simulink model "Main_Sfunction_blocks"  (R2022b)
settings: Solver=FixedStepAuto  StartTime=0.0  StopTime=sim_time-0.02  FixedStep=0.005
undefined symbols (not defined in the file): A_d, B_d, bike_params, C1, C2, counter, D1, D2, D_balancing_inner, D_balancing_outer, DWORK0, DWORK1, DWORK2, e1_max, g, hor_dis, I_balancing_inner, I_balancing_outer, Initial_State, initial_state, initial_state_estimate, k1, k2, Kalman_gain1, Kalman_gain2, lambda, lf, lr, P_balancing_inner, P_balancing_outer, Parameters, pert_deltadot_state, pert_deltadot_state_fun, pert_phidot_state, pert_phidot_state_fun, Psiref, ref_dis, ref_start_idx, T, Ts, v, Xref, Yref
libraries: eeGeneralControl x3, slpidlib x2, simulink x2
(part 1 of 2)
settings Model: PauseTimes=0.16  Creator=Hadi Hajieghrary  LastModifiedBy=levi1
settings SolverCC: MaxConsecutiveMinStep=10  ZeroCrossAlgorithm=Adaptive  AlgebraicLoopSolver=TrustRegion  AutoInsertRateTranBlk=on
settings DebuggingCC: AlgebraicLoopMsg=none  UnconnectedInputMsg=warning  UnconnectedOutputMsg=warning  UnconnectedLineMsg=warning
settings ModelReferenceCC: EnableRefExpFcnMdlSchedulingChecks=on
settings RTWCC: GenCodeOnly=on  DLArmComputeVersion=19.05

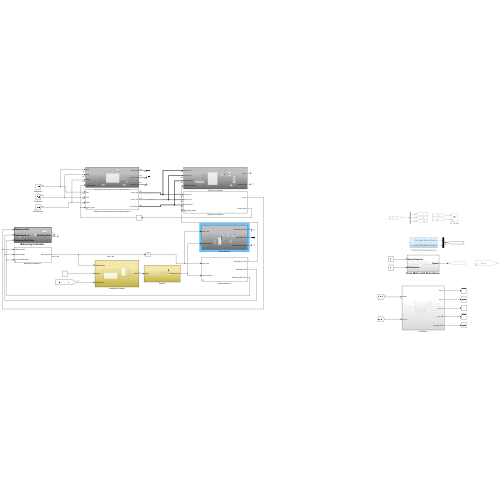
[thumbnail: Simulink's stored preview of the top-level diagram]
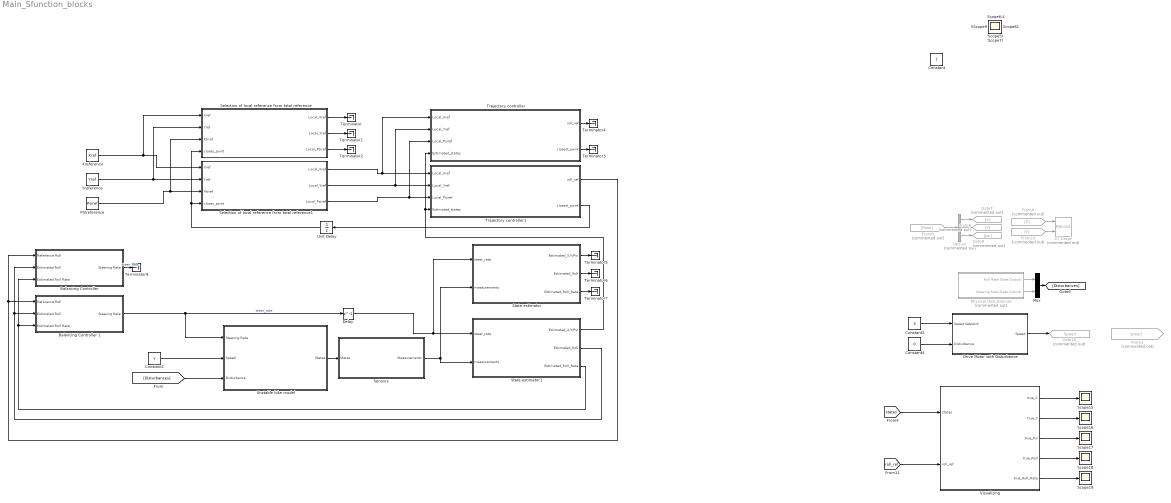
== system Main_Sfunction_blocks ==
  "Balancing Controller " : Subsystem  TreatAsAtomicUnit=on  SystemSampleTime=Ts
      settings: MinAlgLoopOccurrences=on
  Balancing Controller 1 : Subsystem
      mask help: Simulink:masks:GenSFuncDesc_MD
      mask Help: eval('feval(''rtwprivate'',''rtwhelpview'',''rtw_sfcn_block'')');
  Constant1 : Constant  Value=v
  Constant3 : Constant  Value=3
  Constant4 : Constant  Value=0
  Delay : Delay  DelayLength=1  SampleTime=Ts
  Demux : Demux  Commented=on  Outputs=3
  Drive Motor with Disturbance : Subsystem
  From1 : From  Commented=on  GotoTag=Speed  TagVisibility=global
  From10 : From  Commented=on  GotoTag=Y
  From8 : From  Commented=on  GotoTag=Pose
  From9 : From  Commented=on  GotoTag=X
  Goto10 : Goto  Commented=on  GotoTag=Speed  TagVisibility=global
  Goto7 : Goto  Commented=on  GotoTag=X
  Goto8 : Goto  Commented=on  GotoTag=Y
  Goto9 : Goto  Commented=on  GotoTag=psi
  Mux : Mux  Inputs=2
  PSIreference : Constant  Value=Psiref
  Physical Disturbances : Subsystem  Commented=on
  Scope{,1..19} (20 alike) : Scope
  Selection of local reference from total reference : Subsystem
  Selection of local reference from total reference1 : Subsystem
      mask help: Simulink:masks:GenSFuncDesc_MD
      mask Help: eval('feval(''rtwprivate'',''rtwhelpview'',''rtw_sfcn_block'')');
  Sensors : Subsystem
  State estimator : Subsystem
  State estimator1 : Subsystem
      mask help: Simulink:masks:GenSFuncDesc_MD
      mask Help: eval('feval(''rtwprivate'',''rtwhelpview'',''rtw_sfcn_block'')');
  Terminator{,1..8} (9 alike) : Terminator
  Trajectory controller : Subsystem
  Trajectory controller1 : Subsystem
      mask help: Simulink:masks:GenSFuncDesc_MD
      mask Help: eval('feval(''rtwprivate'',''rtwhelpview'',''rtw_sfcn_block'')');
  Unit Delay : UnitDelay  InitialCondition=ref_start_idx  SampleTime=Ts  HasFrameUpgradeWarning=on
  Unstable bike model : Subsystem
  Visualizing : Subsystem
  XY Graph : Record  Commented=on  FileSettingsInternal="{\"entries\":[{\"content\":{\"excelSettings\":{\"content\":{},\"type\":\"Streamout.ExcelSettings\"}},\"type\":\"Streamout.FileSettingStorage\",\"uuid\":\"3eafbd0c-e137-4ee7-8d03-04bb30acaa48\"}],\"packageUris\":[\"http://schema.mathworks.com/mf0/streamout_blocks/R2020a\"],\"version\":\"1.0\"}"  Layout=[1 1]  SignalsInternal="{\"entries\":[{\"content\":{\"signals\":[]},\"type\":\"RecordBlkView.InputSignals\",\"uuid\":\"6eef560f-cd8b-4d38-ad5e-a10ba84618eb\"}],\"packageUris\":[\"http://schema.mathworks.com/mf0/streamout_blocks/R2020a\"],\"version\":\"1.0\"}"  VisualizationBindings="{\"xyplotplugin\":{\"info\":[{\"series\":[],\"subplotID\":1}]}}"  CompatibilityTag=XY
  Xreference : Constant  Value=Xref
  Yreference : Constant  Value=Yref
  Constant : Constant  IOType=siggen
  wires:
  From8/1 -> Demux/1
  Demux/1 -> Goto7/1
  Demux/2 -> Goto8/1
  Demux/3 -> Goto9/1
  From10/1 -> XY Graph/2
  From9/1 -> XY Graph/1
  Physical Disturbances/1(Roll Rate State Disturb) -> Mux/1
  Physical Disturbances/2(Steering Rate State Disturb) -> Mux/2
  Mux/1 -> [Disturbances]
  Drive Motor with Disturbance/1(Speed) -> Goto10/1
  Constant3/1 -> Drive Motor with Disturbance/1(Speed Setpoint)
  Constant4/1 -> Drive Motor with Disturbance/2(Disturbance)
  Balancing Controller 1/1(Steering Rate) -> Unstable bike model/1(Steering Rate), Delay/1  "steer_rate"
  [Disturbances] -> Unstable bike model/3(Disturbance)
  [states] -> Visualizing/1(states)
  Visualizing/1(true_X) -> Scope15/1
  Visualizing/2(true_Y) -> Scope16/1
  Visualizing/3(true_Psi) -> Scope17/1
  Visualizing/4(true_Roll) -> Scope18/1
  Visualizing/5(true_Roll_Rate) -> Scope19/1
  [roll_ref] -> Visualizing/2(roll_ref)
  Unstable bike model/1(States) -> Sensors/1(States)
  Constant1/1 -> Unstable bike model/2(Speed)
  Xreference/1 -> Selection of local reference from total reference/1(Xref), Selection of local reference from total reference1/1(Xref)
  Yreference/1 -> Selection of local reference from total reference/2(Yref), Selection of local reference from total reference1/2(Yref)
  PSIreference/1 -> Selection of local reference from total reference/3(Psiref), Selection of local reference from total reference1/3(Psiref)
  Selection of local reference from total reference1/1(Local_Xref) -> Trajectory controller/1(Local_Xref), Trajectory controller1/1(Local_Xref)
  Selection of local reference from total reference1/2(Local_Yref) -> Trajectory controller/2(Local_Yref), Trajectory controller1/2(Local_Yref)
  Selection of local reference from total reference1/3(Local_Psiref) -> Trajectory controller/3(Local_Psiref), Trajectory controller1/3(Local_Psiref)
  Trajectory controller1/2(closest_point) -> Unit Delay/1
  Unit Delay/1 -> Selection of local reference from total reference/4(closes_point), Selection of local reference from total reference1/4(closes_point)
  Trajectory controller1/1(roll_ref) -> "Balancing Controller "/1(Reference Roll), Balancing Controller 1/1(Reference Roll)
  Sensors/1(Measurements) -> State estimator1/2(measurements), State estimator/2(measurements)
  Delay/1 -> State estimator1/1(steer_rate), State estimator/1(steer_rate)
  State estimator1/1(Estimated_X/Y/Psi) -> Trajectory controller/4(Estimated_states), Trajectory controller1/4(Estimated_states)
  State estimator1/2(Estimated_Roll) -> "Balancing Controller "/2(Estimated Roll), Balancing Controller 1/2(Estimated Roll)
  State estimator1/3(Estimated_Roll_Rate) -> "Balancing Controller "/3(Estimated Roll Rate), Balancing Controller 1/3(Estimated Roll Rate)
  Selection of local reference from total reference/1(Local_Xref) -> Terminator/1
  Selection of local reference from total reference/3(Local_Psiref) -> Terminator2/1
  Selection of local reference from total reference/2(Local_Yref) -> Terminator1/1
  Trajectory controller/1(roll_ref) -> Terminator4/1
  Trajectory controller/2(closest_point) -> Terminator3/1
  State estimator/1(Estimated_X/Y/Psi) -> Terminator5/1
  State estimator/3(Estimated_Roll_Rate) -> Terminator7/1
  State estimator/2(Estimated_Roll) -> Terminator6/1
  "Balancing Controller "/1(Steering Rate) -> Terminator8/1  "steer_rate"

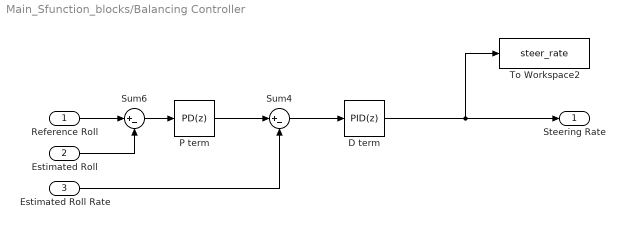
== system Main_Sfunction_blocks/Balancing Controller  ==
  Reference Roll : Inport
  Estimated Roll : Inport  Port=2
  Estimated Roll Rate : Inport  Port=3
  D term : slpidlib/PID Controller  Controller=PID  Form=Parallel  TimeDomain=Discrete-time  UseExternalTs=off  SampleTime=Ts  IntegratorMethod=Forward Euler  FilterMethod=Forward Euler  ControllerParametersSource=internal  P=P_balancing_inner  I=I_balancing_inner  UseKiTs=off  D=D_balancing_inner  N=100  UseFilter=off  TunerSelectOption=Transfer Function Based (PID Tuner App)  InitialConditionSource=internal  InitialConditionForIntegrator=0  InitialConditionForFilter=0  DifferentiatorICPrevScaledInput=0  ExternalReset=none  TrackingMode=off  Kt=1  LimitOutput=off  SatLimitsSource=internal  UpperSaturationLimit=inf  LowerSaturationLimit=-inf  LinearizeAsGain=on  AntiWindupMode=none  Kb=1  LimitIntegrator=off  UpperIntegratorSaturationLimit=inf  LowerIntegratorSaturationLimit=-inf  POutMin=[]  POutMax=[]  IOutMin=[]  IOutMax=[]  DOutMin=[]  DOutMax=[]  NOutMin=[]  NOutMax=[]  SumOutMin=[]  SumOutMax=[]  SaturationOutMin=[]  SaturationOutMax=[]  PParamMin=[]  PParamMax=[]  IParamMin=[]  IParamMax=[]  DParamMin=[]  DParamMax=[]  NParamMin=[]  NParamMax=[]  KbParamMin=[]  KbParamMax=[]  KtParamMin=[]  KtParamMax=[]  KbOutMin=[]  KbOutMax=[]  KtOutMin=[]  KtOutMax=[]  IntegratorOutMin=[]  IntegratorOutMax=[]  FilterOutMin=[]  FilterOutMax=[]  SumI1OutMin=[]  SumI1OutMax=[]  SumI2OutMin=[]  SumI2OutMax=[]  SumI3OutMin=[]  SumI3OutMax=[]  SumI4OutMin=[]  SumI4OutMax=[]  SumDOutMin=[]  SumDOutMax=[]  DifferentiatorOutMin=[]  DifferentiatorOutMax=[]  FilterDiffOutCoefMin=[]  FilterDiffOutCoefMax=[]  ReciprocalOutMin=[]  ReciprocalOutMax=[]  SumDenOutMin=[]  SumDenOutMax=[]  SumNumOutMin=[]  SumNumOutMax=[]  DivideOutMin=[]  DivideOutMax=[]  UdiffTsProdOutMin=[]  UdiffTsProdOutMax=[]  NTsProdOutMin=[]  NTsProdOutMax=[]  UintegralTsProdOutMin=[]  UintegralTsProdOutMax=[]  UngainTsProdOutMin=[]  UngainTsProdOutMax=[]  IntegratorContinuousStateAttributes=''  IntegratorStateMustResolveToSignalObject=off  IntegratorRTWStateStorageClass=Auto  FilterContinuousStateAttributes=''  FilterStateMustResolveToSignalObject=off  FilterRTWStateStorageClass=Auto  ParallelPVariant=InternalParameters  IdealPVariant=Disabled  IVariant=InternalParameters  DVariant=InternalParameters  IntegratorVariant=Discrete  SatVariant=Disabled  AWVariant=Passthrough  PCopyVariant=Disabled  TRVariant=Disabled  FdbkBlocksVariant=Forward  IdealPFdbkVariant=Disabled  SatFdbkVariant=Disabled  DerivativeFilterVariant=Differentiator  NVariant=Passthrough  NCopyVariant=Disabled_SignalSpec  FilterICVariant=InternalICsDifferentiator  IntegratorICVariant=InternalICs  ExternalResetVariant=Disabled  TRSumVariant=Passthrough  SumFdbkVariant=Disabled  SumVariant=Sum_PID  TsampFilterVariant=InternalTs  TsampNgainVariant=Passthrough  TsampIntegralVariant=Passthrough  ExternalSaturationOutDataTypeStr=Inherit: Same as second input
  P term : slpidlib/PID Controller  Controller=PD  Form=Parallel  TimeDomain=Discrete-time  UseExternalTs=off  SampleTime=Ts  IntegratorMethod=Forward Euler  FilterMethod=Forward Euler  ControllerParametersSource=internal  P=P_balancing_outer  I=I_balancing_outer  UseKiTs=off  D=D_balancing_outer  N=100  UseFilter=off  TunerSelectOption=Transfer Function Based (PID Tuner App)  InitialConditionSource=internal  InitialConditionForIntegrator=0  InitialConditionForFilter=0  DifferentiatorICPrevScaledInput=0  ExternalReset=none  TrackingMode=off  Kt=1  LimitOutput=off  SatLimitsSource=internal  UpperSaturationLimit=inf  LowerSaturationLimit=-inf  LinearizeAsGain=on  AntiWindupMode=none  Kb=1  LimitIntegrator=off  UpperIntegratorSaturationLimit=inf  LowerIntegratorSaturationLimit=-inf  POutMin=[]  POutMax=[]  IOutMin=[]  IOutMax=[]  DOutMin=[]  DOutMax=[]  NOutMin=[]  NOutMax=[]  SumOutMin=[]  SumOutMax=[]  SaturationOutMin=[]  SaturationOutMax=[]  PParamMin=[]  PParamMax=[]  IParamMin=[]  IParamMax=[]  DParamMin=[]  DParamMax=[]  NParamMin=[]  NParamMax=[]  KbParamMin=[]  KbParamMax=[]  KtParamMin=[]  KtParamMax=[]  KbOutMin=[]  KbOutMax=[]  KtOutMin=[]  KtOutMax=[]  IntegratorOutMin=[]  IntegratorOutMax=[]  FilterOutMin=[]  FilterOutMax=[]  SumI1OutMin=[]  SumI1OutMax=[]  SumI2OutMin=[]  SumI2OutMax=[]  SumI3OutMin=[]  SumI3OutMax=[]  SumI4OutMin=[]  SumI4OutMax=[]  SumDOutMin=[]  SumDOutMax=[]  DifferentiatorOutMin=[]  DifferentiatorOutMax=[]  FilterDiffOutCoefMin=[]  FilterDiffOutCoefMax=[]  ReciprocalOutMin=[]  ReciprocalOutMax=[]  SumDenOutMin=[]  SumDenOutMax=[]  SumNumOutMin=[]  SumNumOutMax=[]  DivideOutMin=[]  DivideOutMax=[]  UdiffTsProdOutMin=[]  UdiffTsProdOutMax=[]  NTsProdOutMin=[]  NTsProdOutMax=[]  UintegralTsProdOutMin=[]  UintegralTsProdOutMax=[]  UngainTsProdOutMin=[]  UngainTsProdOutMax=[]  IntegratorContinuousStateAttributes=''  IntegratorStateMustResolveToSignalObject=off  IntegratorRTWStateStorageClass=Auto  FilterContinuousStateAttributes=''  FilterStateMustResolveToSignalObject=off  FilterRTWStateStorageClass=Auto  ParallelPVariant=InternalParameters  IdealPVariant=Disabled  IVariant=Disabled  DVariant=InternalParameters  IntegratorVariant=Disabled  SatVariant=Disabled  AWVariant=Disabled  PCopyVariant=Disabled  TRVariant=Disabled  FdbkBlocksVariant=Forward  IdealPFdbkVariant=Disabled  SatFdbkVariant=Disabled  DerivativeFilterVariant=Differentiator  NVariant=Passthrough  NCopyVariant=Disabled_SignalSpec  FilterICVariant=InternalICsDifferentiator  IntegratorICVariant=Disabled  ExternalResetVariant=Disabled  TRSumVariant=Passthrough  SumFdbkVariant=Disabled  SumVariant=Sum_PD  TsampFilterVariant=InternalTs  TsampNgainVariant=Passthrough  TsampIntegralVariant=Disabled_SignalSpec  ExternalSaturationOutDataTypeStr=Inherit: Same as second input
  Sum4 : Sum  Inputs=|+-
  Sum6 : Sum  Inputs=|+-
  To Workspace2 : ToWorkspace  VariableName=steer_rate  SaveFormat=Timeseries  SampleTime=-1
  Steering Rate : Outport
  wires:
  Sum4/1 -> D term/1
  Reference Roll/1 -> Sum6/1
  Sum6/1 -> P term/1
  Estimated Roll Rate/1 -> Sum4/2
  P term/1 -> Sum4/1
  D term/1 -> To Workspace2/1, Steering Rate/1
  Estimated Roll/1 -> Sum6/2

== system Main_Sfunction_blocks/Balancing Controller 1 ==
  Reference Roll : Inport
  Estimated Roll : Inport  Port=2
  Estimated Roll Rate : Inport  Port=3
  Balancing Controller _sfcn : S-Function  FunctionName=Balancing_sf  SFunctionModules=""  SFunctionDeploymentMode=off  EnableBusSupport=off  SFcnStateName=DWORK0,DWORK1,DWORK2  mask{rtw_sf_name=Balancing_sf, showVar=off}
      mask prompts: rtw_sf_name "Simulink:masks:GenSFuncName_MP"; showVar "Simulink:masks:GenSFuncShowModuleList_MP"
      mask help: Simulink:masks:GenSFuncDesc_MD
      mask init:
      | displist = '';
      | if ~strcmp(get_param(gcb, 'FunctionName'), rtw_sf_name);
      |   set_param(gcb, 'FunctionName', rtw_sf_name);
      | end
      | % Check if we are generating code
      | rtw_mode = false;
      | if strcmpi(get_param(bdroot(gcb),'SimulationStatus'),'Initializing')
      | 	rtw_mode = strcmpi(get_param(bdroot(gcb),'BuildingRTWCode'),'on') && ...
      | 		~strcmpi(get_param(bdroot(gcb),'TargetStyle'),'SimulationTarget');
      | end
      | if showVar || rtw_mode
      | 	if exist('rtwsfunc') == 2 | exist('rtwsfunc') == 6
      | 		tmplist = rtwsfunc(rtw_sf_name,gcb);
      | 		tmplist = DAStudio.message('Simulink:masks:GenSFuncListOfModules_IC', tmplist);
      | 	elseif showVar
      | 		tmplist1 = DAStudio.message('Simulink:masks:GenSFuncListOfModules_IC', '');
      |         tmplist2 = DAStudio.message('Simulink:masks:GenSFuncNotLicensed_IC');
      |         tmplist = [tmplist1 tmplist2];
      |  	end
      | end
      | if showVar
      |   displist = tmplist;
      | end
      settings: SFcnIsStateOwnerBlock=on
      settings: CopyFcn=|
      | if ~strcmp(get_param(gcb,'Linkstatus'),'none') && ...
      | ~strcmp(get_param(gcb,'Linkstatus'),'implicit')
      |   set_param(gcb,'LinkStatus','none');
      | end
      mask Help: eval('feval(''rtwprivate'',''rtwhelpview'',''rtw_sfcn_block'')');
      mask Display:
      | port_label('input',1,'Reference Roll');
      | port_label('input',2,'Estimated Roll');
      | port_label('input',3,'Estimated Roll Rate');
      | port_label('output',1,'Steering Rate');
  __InputSSForSFun__ : Subsystem
  __OutputSSForSFun__ : Subsystem
  Steering Rate : Outport
  wires:
  __OutputSSForSFun__/1(Steering Rate) -> Steering Rate/1
  Balancing Controller _sfcn/1 -> __OutputSSForSFun__/1(__UniqueInportName__1__)
  __InputSSForSFun__/3(__UniqueOutportName__3__) -> Balancing Controller _sfcn/3
  __InputSSForSFun__/2(__UniqueOutportName__2__) -> Balancing Controller _sfcn/2
  __InputSSForSFun__/1(__UniqueOutportName__1__) -> Balancing Controller _sfcn/1
  Estimated Roll Rate/1 -> __InputSSForSFun__/3(Estimated Roll Rate)
  Estimated Roll/1 -> __InputSSForSFun__/2(Estimated Roll)
  Reference Roll/1 -> __InputSSForSFun__/1(Reference Roll)

== system Main_Sfunction_blocks/Drive Motor with Disturbance ==
  Speed Setpoint : Inport
  Disturbance : Inport  Port=2
  Sum2 : Sum  Inputs=++|
  Transfer Fcn : TransferFcn  Denominator=[2 1]
  Speed : Outport
  wires:
  Sum2/1 -> Speed/1
  Transfer Fcn/1 -> Sum2/2
  Speed Setpoint/1 -> Transfer Fcn/1
  Disturbance/1 -> Sum2/1

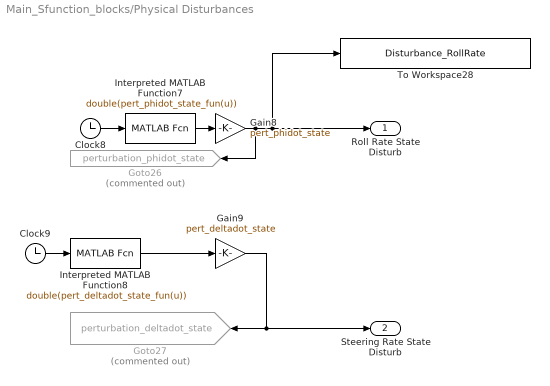
== system Main_Sfunction_blocks/Physical Disturbances ==
  Clock8 : Clock
  Clock9 : Clock
  Gain8 : Gain  Gain=pert_phidot_state
  Gain9 : Gain  Gain=pert_deltadot_state
  Goto26 : Goto  Commented=on  GotoTag=perturbation_phidot_state  TagVisibility=global
  Goto27 : Goto  Commented=on  GotoTag=perturbation_deltadot_state  TagVisibility=global
  Interpreted MATLAB Function7 : MATLABFcn  MATLABFcn=double(pert_phidot_state_fun(u))
  Interpreted MATLAB Function8 : MATLABFcn  MATLABFcn=double(pert_deltadot_state_fun(u))
  To Workspace28 : ToWorkspace  VariableName=Disturbance_RollRate  SaveFormat=Timeseries  SampleTime=-1
  Roll Rate State Disturb : Outport
  Steering Rate State Disturb : Outport  Port=2
  wires:
  Interpreted MATLAB Function7/1 -> Gain8/1
  Clock8/1 -> Interpreted MATLAB Function7/1
  Gain8/1 -> Goto26/1, Roll Rate State Disturb/1, To Workspace28/1
  Interpreted MATLAB Function8/1 -> Gain9/1
  Clock9/1 -> Interpreted MATLAB Function8/1
  Gain9/1 -> Steering Rate State Disturb/1, Goto27/1

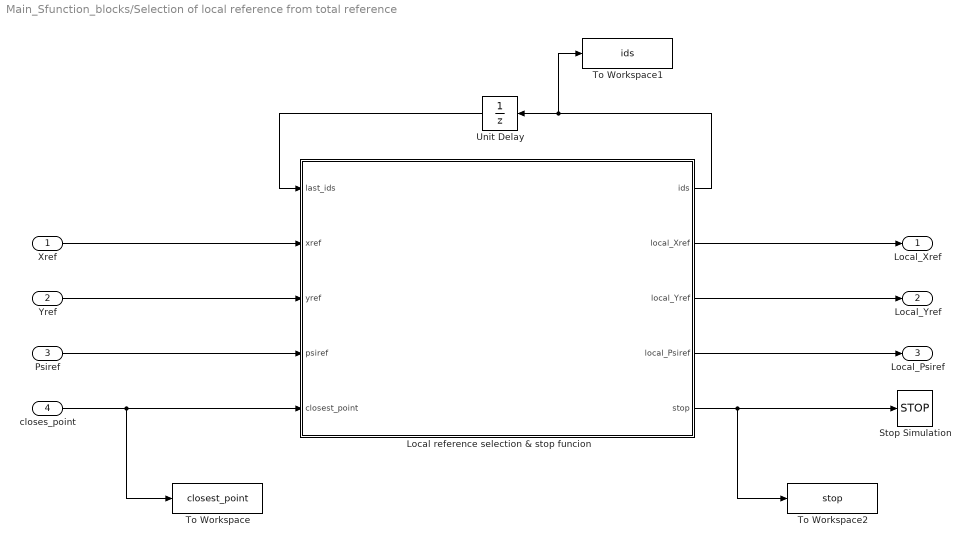
== system Main_Sfunction_blocks/Selection of local reference from total reference ==
  Xref : Inport
  Yref : Inport  Port=2
  Psiref : Inport  Port=3
  closes_point : Inport  Port=4
  Local reference selection & stop funcion : MATLAB Function  TreatAsAtomicUnit=on
  Stop Simulation : Stop
  To Workspace : ToWorkspace  VariableName=closest_point  SaveFormat=Timeseries  SampleTime=-1
  To Workspace1 : ToWorkspace  VariableName=ids  SaveFormat=Timeseries  SampleTime=-1
  To Workspace2 : ToWorkspace  VariableName=stop  SaveFormat=Timeseries  SampleTime=-1
  Unit Delay : UnitDelay  InitialCondition=1  SampleTime=Ts  HasFrameUpgradeWarning=on
  Local_Xref : Outport
  Local_Yref : Outport  Port=2
  Local_Psiref : Outport  Port=3
  wires:
  Local reference selection & stop funcion/1(ids) -> To Workspace1/1, Unit Delay/1
  Unit Delay/1 -> Local reference selection & stop funcion/1(last_ids)
  closes_point/1 -> To Workspace/1, Local reference selection & stop funcion/5(closest_point)
  Xref/1 -> Local reference selection & stop funcion/2(xref)
  Yref/1 -> Local reference selection & stop funcion/3(yref)
  Psiref/1 -> Local reference selection & stop funcion/4(psiref)
  Local reference selection & stop funcion/5(stop) -> To Workspace2/1, Stop Simulation/1
  Local reference selection & stop funcion/2(local_Xref) -> Local_Xref/1
  Local reference selection & stop funcion/3(local_Yref) -> Local_Yref/1
  Local reference selection & stop funcion/4(local_Psiref) -> Local_Psiref/1

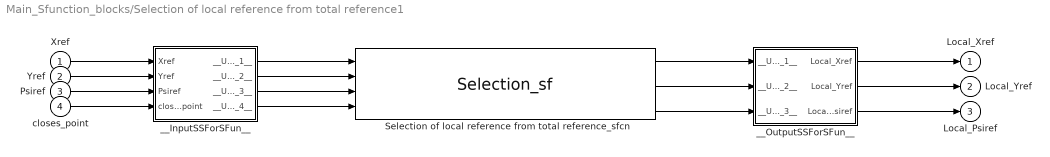
== system Main_Sfunction_blocks/Selection of local reference from total reference1 ==
  Xref : Inport
  Yref : Inport  Port=2
  Psiref : Inport  Port=3
  closes_point : Inport  Port=4
  Selection of local reference from total reference_sfcn : S-Function  FunctionName=Selection_sf  SFunctionModules=""  SFunctionDeploymentMode=off  EnableBusSupport=off  SFcnStateName=DWORK0  mask{rtw_sf_name=Selection_sf, showVar=off}
      mask prompts: rtw_sf_name "Simulink:masks:GenSFuncName_MP"; showVar "Simulink:masks:GenSFuncShowModuleList_MP"
      mask help: Simulink:masks:GenSFuncDesc_MD
      mask init: same as Main_Sfunction_blocks/Balancing Controller 1/Balancing Controller _sfcn
      settings: SFcnIsStateOwnerBlock=on
      settings: CopyFcn=|
      | if ~strcmp(get_param(gcb,'Linkstatus'),'none') && ...
      | ~strcmp(get_param(gcb,'Linkstatus'),'implicit')
      |   set_param(gcb,'LinkStatus','none');
      | end
      mask Help: eval('feval(''rtwprivate'',''rtwhelpview'',''rtw_sfcn_block'')');
      mask Display:
      | port_label('input',1,'Xref');
      | port_label('input',2,'Yref');
      | port_label('input',3,'Psiref');
      | port_label('input',4,'closes_point');
      | port_label('output',1,'Local_Xref');
      | port_label('output',2,'Local_Yref');
      | port_label('output',3,'Local_Psiref');
  __InputSSForSFun__ : Subsystem
  __OutputSSForSFun__ : Subsystem
  Local_Xref : Outport
  Local_Yref : Outport  Port=2
  Local_Psiref : Outport  Port=3
  wires:
  Xref/1 -> __InputSSForSFun__/1(Xref)
  Yref/1 -> __InputSSForSFun__/2(Yref)
  Psiref/1 -> __InputSSForSFun__/3(Psiref)
  closes_point/1 -> __InputSSForSFun__/4(closes_point)
  __InputSSForSFun__/1(__UniqueOutportName__1__) -> Selection of local reference from total reference_sfcn/1
  __InputSSForSFun__/2(__UniqueOutportName__2__) -> Selection of local reference from total reference_sfcn/2
  __InputSSForSFun__/3(__UniqueOutportName__3__) -> Selection of local reference from total reference_sfcn/3
  __InputSSForSFun__/4(__UniqueOutportName__4__) -> Selection of local reference from total reference_sfcn/4
  Selection of local reference from total reference_sfcn/1 -> __OutputSSForSFun__/1(__UniqueInportName__1__)
  Selection of local reference from total reference_sfcn/2 -> __OutputSSForSFun__/2(__UniqueInportName__2__)
  Selection of local reference from total reference_sfcn/3 -> __OutputSSForSFun__/3(__UniqueInportName__3__)
  __OutputSSForSFun__/1(Local_Xref) -> Local_Xref/1
  __OutputSSForSFun__/2(Local_Yref) -> Local_Yref/1
  __OutputSSForSFun__/3(Local_Psiref) -> Local_Psiref/1

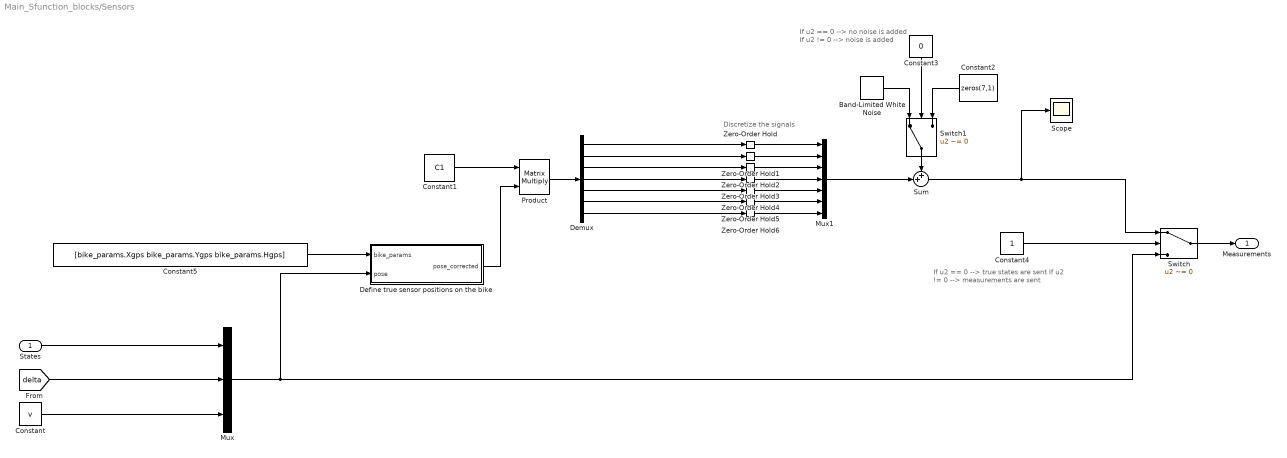
== system Main_Sfunction_blocks/Sensors ==
  note: Discretize the signals
  note: If u2 == 0 --> no noise is added
      | If u2 != 0 --> noise is added
  note: If u2 == 0 --> true states are sent
      | If u2 != 0 --> measurements are sent
  States : Inport
  Band-Limited White Noise : simulink/Sources/Band-Limited White Noise  Cov=ones(7,1)*1e-3  Ts=Ts  seed=[23341]
  Constant : Constant  Value=v
  Constant1 : Constant  Value=C1
  Constant2 : Constant  Value=zeros(7,1)
  Constant3 : Constant  Value=0
  Constant4 : Constant
  Constant5 : Constant  Value=[bike_params.Xgps bike_params.Ygps bike_params.Hgps]
  Define true sensor positions on the bike : MATLAB Function  TreatAsAtomicUnit=on
  Demux : Demux  Outputs=7
  Mux : Mux  Inputs=3
  Mux1 : Mux  Inputs=7
  Product : Product  Multiplication=Matrix(*)
  Scope : Scope
  Sum : Sum  Inputs=++|
  Switch : Switch  Criteria=u2 ~= 0  SaturateOnIntegerOverflow=off  InputSameDT=off
  Switch1 : Switch  Criteria=u2 ~= 0  SaturateOnIntegerOverflow=off  InputSameDT=off
  Zero-Order Hold : ZeroOrderHold  SampleTime=10*Ts
  Zero-Order Hold1 : ZeroOrderHold  SampleTime=10*Ts
  Zero-Order Hold{2..6} (5 alike) : ZeroOrderHold  SampleTime=Ts
  Measurements : Outport
  wires:
  Constant/1 -> Mux/3
  [delta] -> Mux/2
  States/1 -> Mux/1
  Switch/1 -> Measurements/1
  Mux/1 -> Switch/3, Define true sensor positions on the bike/2(pose)
  Constant4/1 -> Switch/2
  Constant1/1 -> Product/1
  Switch1/1 -> Sum/1
  Band-Limited White Noise/1 -> Switch1/1
  Constant2/1 -> Switch1/3
  Constant3/1 -> Switch1/2
  Mux1/1 -> Sum/2
  Product/1 -> Demux/1
  Demux/2 -> Zero-Order Hold1/1
  Demux/3 -> Zero-Order Hold2/1
  Demux/4 -> Zero-Order Hold3/1
  Demux/5 -> Zero-Order Hold4/1
  Demux/6 -> Zero-Order Hold5/1
  Demux/7 -> Zero-Order Hold6/1
  Zero-Order Hold/1 -> Mux1/1
  Zero-Order Hold1/1 -> Mux1/2
  Zero-Order Hold2/1 -> Mux1/3
  Zero-Order Hold3/1 -> Mux1/4
  Zero-Order Hold4/1 -> Mux1/5
  Zero-Order Hold5/1 -> Mux1/6
  Zero-Order Hold6/1 -> Mux1/7
  Sum/1 -> Scope/1, Switch/1
  Demux/1 -> Zero-Order Hold/1
  Define true sensor positions on the bike/1(pose_corrected) -> Product/2
  Constant5/1 -> Define true sensor positions on the bike/1(bike_params)

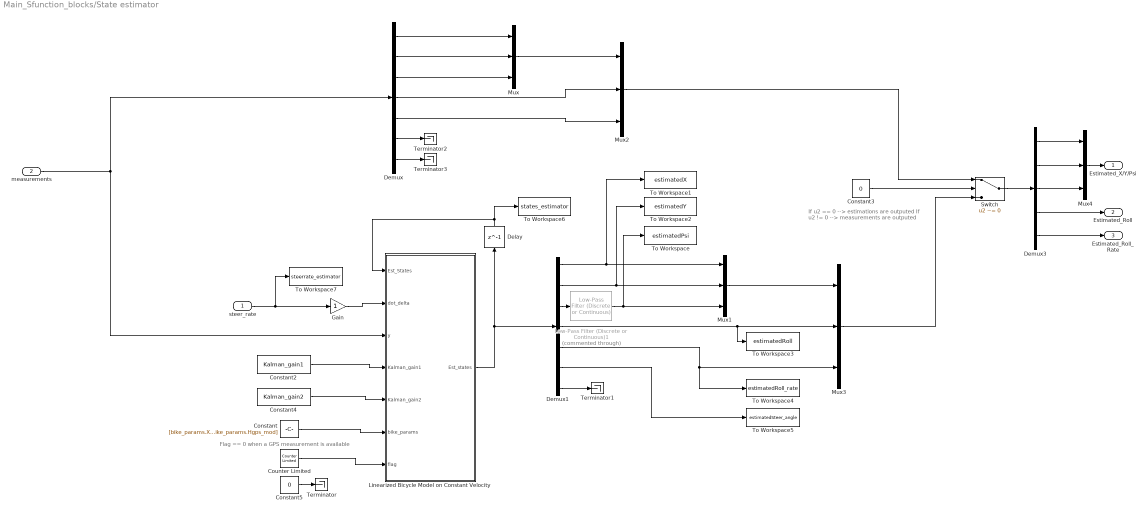
== system Main_Sfunction_blocks/State estimator ==
  note: Flag == 0 when a GPS measurement is available
  note: If u2 == 0 --> estimations are outputed
      | If u2 != 0 --> measurements are outputed
  steer_rate : Inport
  measurements : Inport  Port=2
  Constant : Constant  Value=[bike_params.Xgps_mod bike_params.Ygps_mod bike_params.Hgps_mod]
  Constant2 : Constant  Value=Kalman_gain1  SampleTime=Ts
  Constant3 : Constant  Value=0
  Constant4 : Constant  Value=Kalman_gain2  SampleTime=Ts
  Constant5 : Constant  Value=0
  Counter Limited : simulink/Sources/Counter Limited  uplimit=counter  tsamp=Ts
  Delay : Delay  DelayLength=1  InitialCondition=[initial_state_estimate.x initial_state_estimate.y initial_state_estimate.heading initial_state.roll initial_state.roll_rate initial_state.steering v]  SampleTime=Ts
  Demux : Demux  Outputs=7
  Demux1 : Demux  Outputs=7
  Demux3 : Demux  Outputs=5
  Gain : Gain
  Linearized Bicycle Model on Constant Velocity : MATLAB Function  TreatAsAtomicUnit=on
  Low-Pass Filter (Discrete or Continuous)1 : eeGeneralControl/Low-Pass Filter (Discrete or Continuous)  Commented=through  K=1  T=1  B=inf  A=-inf  init_option=Inherited from block input  x0=0  Ts=Ts
  Mux{,1..4} (5 alike) : Mux  Inputs=3
  Switch : Switch  Criteria=u2 ~= 0  SaturateOnIntegerOverflow=off  InputSameDT=off
  Terminator{,1..3} (4 alike) : Terminator
  To Workspace : ToWorkspace  VariableName=estimatedPsi  SaveFormat=Timeseries  SampleTime=-1
  To Workspace1 : ToWorkspace  VariableName=estimatedX  SaveFormat=Timeseries  SampleTime=-1
  To Workspace2 : ToWorkspace  VariableName=estimatedY  SaveFormat=Timeseries  SampleTime=-1
  To Workspace3 : ToWorkspace  VariableName=estimatedRoll  SaveFormat=Timeseries  SampleTime=-1
  To Workspace4 : ToWorkspace  VariableName=estimatedRoll_rate  SaveFormat=Timeseries  SampleTime=-1
  To Workspace5 : ToWorkspace  VariableName=estimatedSteer_angle  SaveFormat=Timeseries  SampleTime=-1
  To Workspace6 : ToWorkspace  VariableName=states_estimator  SaveFormat=Timeseries  SampleTime=-1
  To Workspace7 : ToWorkspace  VariableName=steerrate_estimator  SaveFormat=Timeseries  SampleTime=-1
  Estimated_X/Y/Psi : Outport  VectorParamsAs1DForOutWhenUnconnected=off
  Estimated_Roll : Outport  Port=2  VectorParamsAs1DForOutWhenUnconnected=off
  Estimated_Roll_Rate : Outport  Port=3  VectorParamsAs1DForOutWhenUnconnected=off
  wires:
  Demux/3 -> Mux/3
  Linearized Bicycle Model on Constant Velocity/1(Est_states) -> Delay/1, Demux1/1
  Gain/1 -> Linearized Bicycle Model on Constant Velocity/2(dot_delta)
  Demux1/6 -> To Workspace5/1
  Demux1/5 -> Mux3/3, To Workspace4/1
  Delay/1 -> Linearized Bicycle Model on Constant Velocity/1(Est_States), To Workspace6/1
  steer_rate/1 -> To Workspace7/1, Gain/1
  Demux1/2 -> To Workspace2/1, Mux1/2
  measurements/1 -> Linearized Bicycle Model on Constant Velocity/3(y), Demux/1
  Demux/1 -> Mux/1
  Demux1/3 -> Low-Pass Filter (Discrete or Continuous)1/1
  Demux1/1 -> Mux1/1, To Workspace1/1
  Demux/2 -> Mux/2
  Demux1/7 -> Terminator1/1
  Demux/7 -> Terminator3/1
  Demux/6 -> Terminator2/1
  Mux/1 -> Mux2/1
  Mux2/1 -> Switch/1
  Mux3/1 -> Switch/3
  Constant3/1 -> Switch/2
  Demux/4 -> Mux2/2
  Demux/5 -> Mux2/3
  Mux1/1 -> Mux3/1
  Demux1/4 -> To Workspace3/1, Mux3/2
  Switch/1 -> Demux3/1
  Demux3/1 -> Mux4/1
  Demux3/2 -> Mux4/2
  Demux3/3 -> Mux4/3
  Mux4/1 -> Estimated_X/Y/Psi/1
  Demux3/4 -> Estimated_Roll/1
  Demux3/5 -> Estimated_Roll_Rate/1
  Constant2/1 -> Linearized Bicycle Model on Constant Velocity/4(Kalman_gain1)
  Constant4/1 -> Linearized Bicycle Model on Constant Velocity/5(Kalman_gain2)
  Counter Limited/1 -> Linearized Bicycle Model on Constant Velocity/7(flag)
  Low-Pass Filter (Discrete or Continuous)1/1 -> To Workspace/1, Mux1/3
  Constant5/1 -> Terminator/1
  Constant/1 -> Linearized Bicycle Model on Constant Velocity/6(bike_params)

== system Main_Sfunction_blocks/State estimator1 ==
  steer_rate : Inport
  measurements : Inport  Port=2
  State estimator_sfcn : S-Function  FunctionName=State_sf  SFunctionModules=""  SFunctionDeploymentMode=off  EnableBusSupport=off  SFcnStateName=DWORK0,DWORK1  mask{rtw_sf_name=State_sf, showVar=off}
      mask prompts: rtw_sf_name "Simulink:masks:GenSFuncName_MP"; showVar "Simulink:masks:GenSFuncShowModuleList_MP"
      mask help: Simulink:masks:GenSFuncDesc_MD
      mask init: same as Main_Sfunction_blocks/Balancing Controller 1/Balancing Controller _sfcn
      settings: SFcnIsStateOwnerBlock=on
      settings: CopyFcn=|
      | if ~strcmp(get_param(gcb,'Linkstatus'),'none') && ...
      | ~strcmp(get_param(gcb,'Linkstatus'),'implicit')
      |   set_param(gcb,'LinkStatus','none');
      | end
      mask Help: eval('feval(''rtwprivate'',''rtwhelpview'',''rtw_sfcn_block'')');
      mask Display:
      | port_label('input',1,'steer_rate');
      | port_label('input',2,'measurements');
      | port_label('output',1,'Estimated_X/Y/Psi');
      | port_label('output',2,'Estimated_Roll');
      | port_label('output',3,'Estimated_Roll_Rate');
  __InputSSForSFun__ : Subsystem
  __OutputSSForSFun__ : Subsystem
  Estimated_X/Y/Psi : Outport  VectorParamsAs1DForOutWhenUnconnected=off
  Estimated_Roll : Outport  Port=2  VectorParamsAs1DForOutWhenUnconnected=off
  Estimated_Roll_Rate : Outport  Port=3  VectorParamsAs1DForOutWhenUnconnected=off
  wires:
  __OutputSSForSFun__/3(Estimated_Roll_Rate) -> Estimated_Roll_Rate/1
  __OutputSSForSFun__/2(Estimated_Roll) -> Estimated_Roll/1
  __OutputSSForSFun__/1(Estimated_X/Y/Psi) -> Estimated_X/Y/Psi/1
  State estimator_sfcn/3 -> __OutputSSForSFun__/3(__UniqueInportName__3__)
  State estimator_sfcn/2 -> __OutputSSForSFun__/2(__UniqueInportName__2__)
  State estimator_sfcn/1 -> __OutputSSForSFun__/1(__UniqueInportName__1__)
  __InputSSForSFun__/2(__UniqueOutportName__2__) -> State estimator_sfcn/2
  __InputSSForSFun__/1(__UniqueOutportName__1__) -> State estimator_sfcn/1
  measurements/1 -> __InputSSForSFun__/2(measurements)
  steer_rate/1 -> __InputSSForSFun__/1(steer_rate)

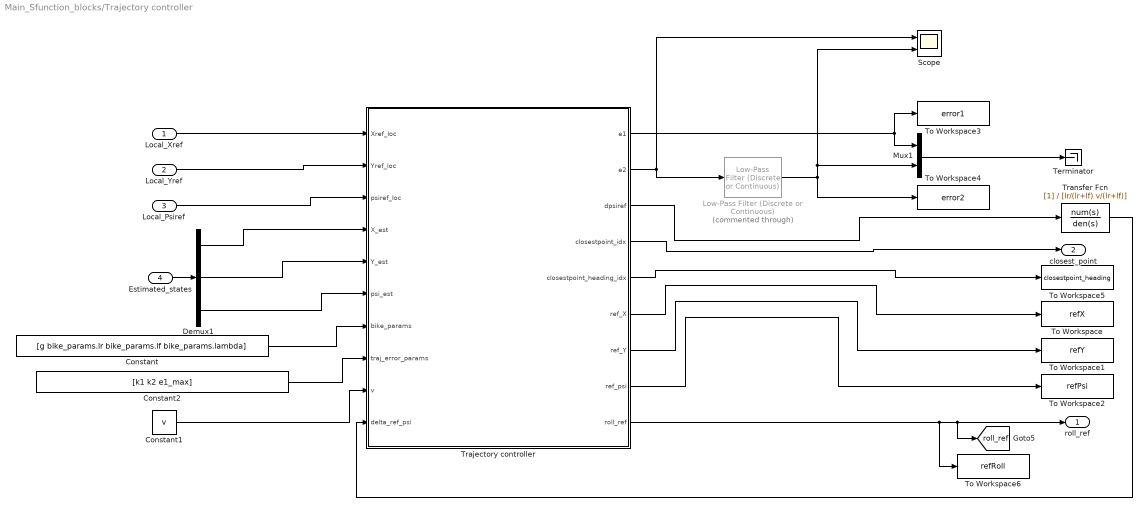
== system Main_Sfunction_blocks/Trajectory controller ==
  Local_Xref : Inport
  Local_Yref : Inport  Port=2
  Local_Psiref : Inport  Port=3
  Estimated_states : Inport  Port=4
  Constant : Constant  Value=[g bike_params.lr bike_params.lf bike_params.lambda]
  Constant1 : Constant  Value=v
  Constant2 : Constant  Value=[k1 k2 e1_max]
  Demux1 : Demux  Outputs=3
  Low-Pass Filter (Discrete or Continuous) : eeGeneralControl/Low-Pass Filter (Discrete or Continuous)  Commented=through  K=1  T=1  B=inf  A=-inf  init_option=Inherited from block input  x0=0  Ts=Ts
  Mux1 : Mux  Inputs=2
  Scope : Scope  NumInputPorts=2
  Terminator : Terminator
  To Workspace : ToWorkspace  VariableName=refX  SaveFormat=Timeseries  SampleTime=-1
  To Workspace1 : ToWorkspace  VariableName=refY  SaveFormat=Timeseries  SampleTime=-1
  To Workspace2 : ToWorkspace  VariableName=refPsi  SaveFormat=Timeseries  SampleTime=-1
  To Workspace3 : ToWorkspace  VariableName=error1  SaveFormat=Timeseries  SampleTime=-1
  To Workspace4 : ToWorkspace  VariableName=error2  SaveFormat=Timeseries  SampleTime=-1
  To Workspace5 : ToWorkspace  VariableName=closestpoint_heading  SaveFormat=Timeseries  SampleTime=-1
  To Workspace6 : ToWorkspace  VariableName=refRoll  SaveFormat=Timeseries  SampleTime=-1
  Trajectory controller : MATLAB Function  TreatAsAtomicUnit=on
  Transfer Fcn : TransferFcn  Denominator=[lr/(lr+lf) v/(lr+lf)]
  roll_ref : Outport
  closest_point : Outport  Port=2
  tag scope: roll_ref=global
  wires:
  Demux1/3 -> Trajectory controller/6(psi_est)
  Trajectory controller/4(closestpoint_idx) -> closest_point/1
  Trajectory controller/5(closestpoint_heading_idx) -> To Workspace5/1
  Estimated_states/1 -> Demux1/1
  Low-Pass Filter (Discrete or Continuous)/1 -> Mux1/2, Scope/2, To Workspace4/1
  Local_Xref/1 -> Trajectory controller/1(Xref_loc)
  Local_Psiref/1 -> Trajectory controller/3(psiref_loc)
  Mux1/1 -> Terminator/1
  Trajectory controller/3(dpsiref) -> Transfer Fcn/1
  Trajectory controller/7(ref_Y) -> To Workspace1/1
  Trajectory controller/2(e2) -> Low-Pass Filter (Discrete or Continuous)/1, Scope/1
  Demux1/2 -> Trajectory controller/5(Y_est)
  Local_Yref/1 -> Trajectory controller/2(Yref_loc)
  Demux1/1 -> Trajectory controller/4(X_est)
  Trajectory controller/6(ref_X) -> To Workspace/1
  Trajectory controller/8(ref_psi) -> To Workspace2/1
  Trajectory controller/1(e1) -> To Workspace3/1, Mux1/1
  Constant1/1 -> Trajectory controller/9(v)
  Constant/1 -> Trajectory controller/7(bike_params)
  Constant2/1 -> Trajectory controller/8(traj_error_params)
  Trajectory controller/9(roll_ref) -> To Workspace6/1, [roll_ref], roll_ref/1
  Transfer Fcn/1 -> Trajectory controller/10(delta_ref_psi)

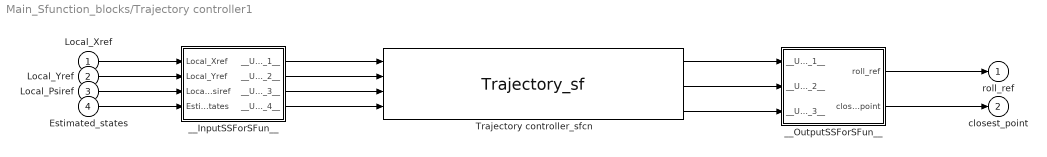
== system Main_Sfunction_blocks/Trajectory controller1 ==
  Local_Xref : Inport
  Local_Yref : Inport  Port=2
  Local_Psiref : Inport  Port=3
  Estimated_states : Inport  Port=4
  Trajectory controller_sfcn : S-Function  FunctionName=Trajectory_sf  SFunctionModules=""  SFunctionDeploymentMode=off  EnableBusSupport=off  mask{rtw_sf_name=Trajectory_sf, showVar=off}
      mask prompts: rtw_sf_name "Simulink:masks:GenSFuncName_MP"; showVar "Simulink:masks:GenSFuncShowModuleList_MP"
      mask help: Simulink:masks:GenSFuncDesc_MD
      mask init: same as Main_Sfunction_blocks/Balancing Controller 1/Balancing Controller _sfcn
      settings: CopyFcn=|
      | if ~strcmp(get_param(gcb,'Linkstatus'),'none') && ...
      | ~strcmp(get_param(gcb,'Linkstatus'),'implicit')
      |   set_param(gcb,'LinkStatus','none');
      | end
      mask Help: eval('feval(''rtwprivate'',''rtwhelpview'',''rtw_sfcn_block'')');
      mask Display:
      | port_label('input',1,'Local_Xref');
      | port_label('input',2,'Local_Yref');
      | port_label('input',3,'Local_Psiref');
      | port_label('input',4,'Estimated_states');
      | port_label('output',1,'roll_ref');
      | port_label('output',2,'closest_point');
      | port_label('output',3,'Outport1');
  __InputSSForSFun__ : Subsystem
  __OutputSSForSFun__ : Subsystem
  roll_ref : Outport
  closest_point : Outport  Port=2
  wires:
  __OutputSSForSFun__/2(closest_point) -> closest_point/1
  __OutputSSForSFun__/1(roll_ref) -> roll_ref/1
  Trajectory controller_sfcn/3 -> __OutputSSForSFun__/3(__UniqueInportName__3__)
  Trajectory controller_sfcn/2 -> __OutputSSForSFun__/2(__UniqueInportName__2__)
  Trajectory controller_sfcn/1 -> __OutputSSForSFun__/1(__UniqueInportName__1__)
  __InputSSForSFun__/4(__UniqueOutportName__4__) -> Trajectory controller_sfcn/4
  __InputSSForSFun__/3(__UniqueOutportName__3__) -> Trajectory controller_sfcn/3
  __InputSSForSFun__/2(__UniqueOutportName__2__) -> Trajectory controller_sfcn/2
  __InputSSForSFun__/1(__UniqueOutportName__1__) -> Trajectory controller_sfcn/1
  Estimated_states/1 -> __InputSSForSFun__/4(Estimated_states)
  Local_Psiref/1 -> __InputSSForSFun__/3(Local_Psiref)
  Local_Yref/1 -> __InputSSForSFun__/2(Local_Yref)
  Local_Xref/1 -> __InputSSForSFun__/1(Local_Xref)

== system Main_Sfunction_blocks/Unstable bike model ==
  Steering Rate : Inport
  Speed : Inport  Port=2
  Disturbance : Inport  Port=3
  Mux : Mux  Inputs=2
  Mux1 : Mux  Inputs=2
  Nonlinear Bicycle model : Subsystem
  Track bycicle pose : Subsystem
  States : Outport
  tag scope: states=global
  wires:
  Steering Rate/1 -> Nonlinear Bicycle model/2(Steering Rate)
  Nonlinear Bicycle model/2(Roll) -> Mux1/1
  Nonlinear Bicycle model/3(Roll Rate) -> Mux1/2
  Mux/1 -> States/1, [states]
  Mux1/1 -> Mux/2
  Speed/1 -> Track bycicle pose/1(Speed), Nonlinear Bicycle model/1(Speed)
  Disturbance/1 -> Nonlinear Bicycle model/3(Disturbances (phi_dot; delta_dot))
  Nonlinear Bicycle model/1(Steer angle) -> Track bycicle pose/2(Steer angle)
  Track bycicle pose/1(Pose) -> Mux/1

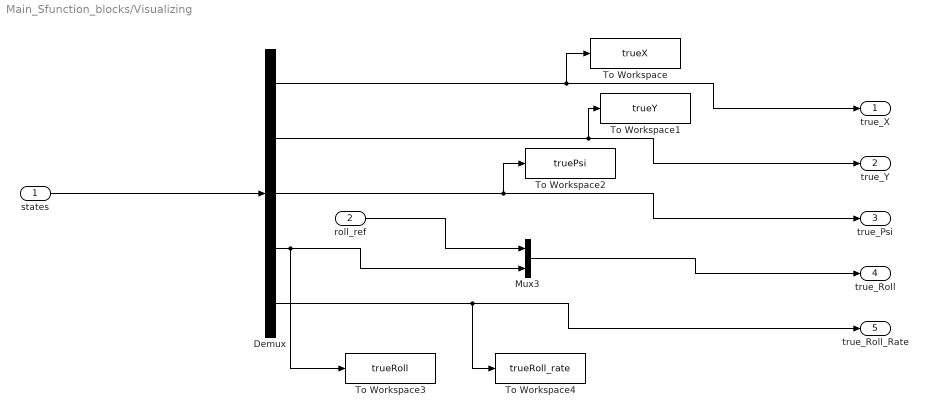
== system Main_Sfunction_blocks/Visualizing ==
  states : Inport
  roll_ref : Inport  Port=2
  Demux : Demux  Outputs=5
  Mux3 : Mux  Inputs=2
  To Workspace : ToWorkspace  VariableName=trueX  SaveFormat=Timeseries  SampleTime=-1
  To Workspace1 : ToWorkspace  VariableName=trueY  SaveFormat=Timeseries  SampleTime=-1
  To Workspace2 : ToWorkspace  VariableName=truePsi  SaveFormat=Timeseries  SampleTime=-1
  To Workspace3 : ToWorkspace  VariableName=trueRoll  SaveFormat=Timeseries  SampleTime=-1
  To Workspace4 : ToWorkspace  VariableName=trueRoll_rate  SaveFormat=Timeseries  SampleTime=-1
  true_X : Outport
  true_Y : Outport  Port=2
  true_Psi : Outport  Port=3
  true_Roll : Outport  Port=4
  true_Roll_Rate : Outport  Port=5
  wires:
  states/1 -> Demux/1
  Demux/1 -> true_X/1, To Workspace/1
  Demux/3 -> To Workspace2/1, true_Psi/1
  roll_ref/1 -> Mux3/1
  Demux/4 -> To Workspace3/1, Mux3/2
  Mux3/1 -> true_Roll/1
  Demux/5 -> To Workspace4/1, true_Roll_Rate/1
  Demux/2 -> To Workspace1/1, true_Y/1

== system Main_Sfunction_blocks/Balancing Controller 1/__InputSSForSFun__ ==
  Reference Roll : Inport
  Estimated Roll : Inport  Port=2
  Estimated Roll Rate : Inport  Port=3
  __UniqueOutportName__1__ : Outport
  __UniqueOutportName__2__ : Outport  Port=2
  __UniqueOutportName__3__ : Outport  Port=3
  wires:
  Estimated Roll Rate/1 -> __UniqueOutportName__3__/1
  Estimated Roll/1 -> __UniqueOutportName__2__/1
  Reference Roll/1 -> __UniqueOutportName__1__/1

== system Main_Sfunction_blocks/Balancing Controller 1/__OutputSSForSFun__ ==
  __UniqueInportName__1__ : Inport
  Steering Rate : Outport
  wires:
  __UniqueInportName__1__/1 -> Steering Rate/1

== system Main_Sfunction_blocks/Selection of local reference from total reference1/__InputSSForSFun__ ==
  Xref : Inport
  Yref : Inport  Port=2
  Psiref : Inport  Port=3
  closes_point : Inport  Port=4
  __UniqueOutportName__1__ : Outport
  __UniqueOutportName__2__ : Outport  Port=2
  __UniqueOutportName__3__ : Outport  Port=3
  __UniqueOutportName__4__ : Outport  Port=4
  wires:
  Xref/1 -> __UniqueOutportName__1__/1
  Yref/1 -> __UniqueOutportName__2__/1
  Psiref/1 -> __UniqueOutportName__3__/1
  closes_point/1 -> __UniqueOutportName__4__/1

== system Main_Sfunction_blocks/Selection of local reference from total reference1/__OutputSSForSFun__ ==
  __UniqueInportName__1__ : Inport
  __UniqueInportName__2__ : Inport  Port=2
  __UniqueInportName__3__ : Inport  Port=3
  Local_Xref : Outport
  Local_Yref : Outport  Port=2
  Local_Psiref : Outport  Port=3
  wires:
  __UniqueInportName__1__/1 -> Local_Xref/1  "local_Xref"
  __UniqueInportName__2__/1 -> Local_Yref/1  "local_Yref"
  __UniqueInportName__3__/1 -> Local_Psiref/1  "local_Psiref"

== system Main_Sfunction_blocks/State estimator1/__InputSSForSFun__ ==
  steer_rate : Inport
  measurements : Inport  Port=2
  __UniqueOutportName__1__ : Outport
  __UniqueOutportName__2__ : Outport  Port=2
  wires:
  measurements/1 -> __UniqueOutportName__2__/1
  steer_rate/1 -> __UniqueOutportName__1__/1

== system Main_Sfunction_blocks/State estimator1/__OutputSSForSFun__ ==
  __UniqueInportName__1__ : Inport
  __UniqueInportName__2__ : Inport  Port=2
  __UniqueInportName__3__ : Inport  Port=3
  Estimated_X/Y/Psi : Outport  VectorParamsAs1DForOutWhenUnconnected=off
  Estimated_Roll : Outport  Port=2  VectorParamsAs1DForOutWhenUnconnected=off
  Estimated_Roll_Rate : Outport  Port=3  VectorParamsAs1DForOutWhenUnconnected=off
  wires:
  __UniqueInportName__3__/1 -> Estimated_Roll_Rate/1
  __UniqueInportName__2__/1 -> Estimated_Roll/1
  __UniqueInportName__1__/1 -> Estimated_X/Y/Psi/1

== system Main_Sfunction_blocks/Trajectory controller1/__InputSSForSFun__ ==
  Local_Xref : Inport
  Local_Yref : Inport  Port=2
  Local_Psiref : Inport  Port=3
  Estimated_states : Inport  Port=4
  __UniqueOutportName__1__ : Outport
  __UniqueOutportName__2__ : Outport  Port=2
  __UniqueOutportName__3__ : Outport  Port=3
  __UniqueOutportName__4__ : Outport  Port=4
  wires:
  Estimated_states/1 -> __UniqueOutportName__4__/1
  Local_Psiref/1 -> __UniqueOutportName__3__/1
  Local_Yref/1 -> __UniqueOutportName__2__/1
  Local_Xref/1 -> __UniqueOutportName__1__/1

== system Main_Sfunction_blocks/Trajectory controller1/__OutputSSForSFun__ ==
  __UniqueInportName__1__ : Inport
  __UniqueInportName__2__ : Inport  Port=2
  __UniqueInportName__3__ : Inport  Port=3
  Terminator : Terminator
  roll_ref : Outport
  closest_point : Outport  Port=2
  wires:
  __UniqueInportName__2__/1 -> closest_point/1  "closestpoint_idx"
  __UniqueInportName__1__/1 -> roll_ref/1  "roll_ref"
  __UniqueInportName__3__/1 -> Terminator/1  "roll_ref"

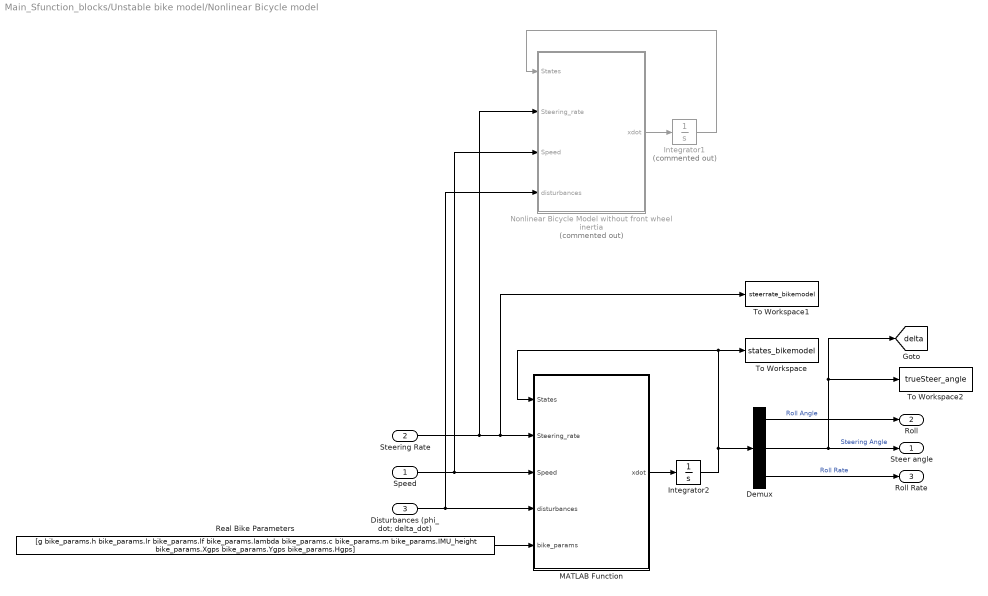
== system Main_Sfunction_blocks/Unstable bike model/Nonlinear Bicycle model ==
  Speed : Inport
  Steering Rate : Inport  Port=2
  Disturbances (phi_dot; delta_dot) : Inport  Port=3
  Demux : Demux  Outputs=3
  Integrator1 : Integrator  Commented=on  InitialCondition=[Initial_State.roll ; Initial_State.steering ; Initial_State.roll_rate]
  Integrator2 : Integrator  InitialCondition=[initial_state.roll ; initial_state.steering ; initial_state.roll_rate]
  MATLAB Function : MATLAB Function  TreatAsAtomicUnit=on
  Nonlinear Bicycle Model without front wheel inertia : MATLAB Function  Commented=on  TreatAsAtomicUnit=on  mask{Parameters=Parameters}
  Real Bike Parameters : Constant  Value=[g bike_params.h bike_params.lr bike_params.lf bike_params.lambda bike_params.c bike_params.m bike_params.IMU_height bike_params.Xgps bike_params.Ygps bike_params.Hgps]  SampleTime=Ts
  To Workspace : ToWorkspace  VariableName=states_bikemodel  SaveFormat=Timeseries  SampleTime=-1
  To Workspace1 : ToWorkspace  VariableName=steerrate_bikemodel  SaveFormat=Timeseries  SampleTime=-1
  To Workspace2 : ToWorkspace  VariableName=trueSteer_angle  SaveFormat=Timeseries  SampleTime=-1
  Steer angle : Outport  VectorParamsAs1DForOutWhenUnconnected=off
  Roll : Outport  Port=2  VectorParamsAs1DForOutWhenUnconnected=off
  Roll Rate : Outport  Port=3  VectorParamsAs1DForOutWhenUnconnected=off
  tag scope: delta=global
  wires:
  Integrator2/1 -> MATLAB Function/1(States), To Workspace/1, Demux/1
  Steering Rate/1 -> Nonlinear Bicycle Model without front wheel inertia/2(Steering_rate), To Workspace1/1, MATLAB Function/2(Steering_rate)
  Disturbances (phi_dot; delta_dot)/1 -> MATLAB Function/4(disturbances), Nonlinear Bicycle Model without front wheel inertia/4(disturbances)
  Real Bike Parameters/1 -> MATLAB Function/5(bike_params)
  Integrator1/1 -> Nonlinear Bicycle Model without front wheel inertia/1(States)
  MATLAB Function/1(xdot) -> Integrator2/1
  Speed/1 -> Nonlinear Bicycle Model without front wheel inertia/3(Speed), MATLAB Function/3(Speed)
  Demux/1 -> Roll/1  "Roll Angle"
  Demux/3 -> Roll Rate/1  "Roll Rate"
  Demux/2 -> To Workspace2/1, [delta], Steer angle/1  "Steering Angle"
  Nonlinear Bicycle Model without front wheel inertia/1(xdot) -> Integrator1/1

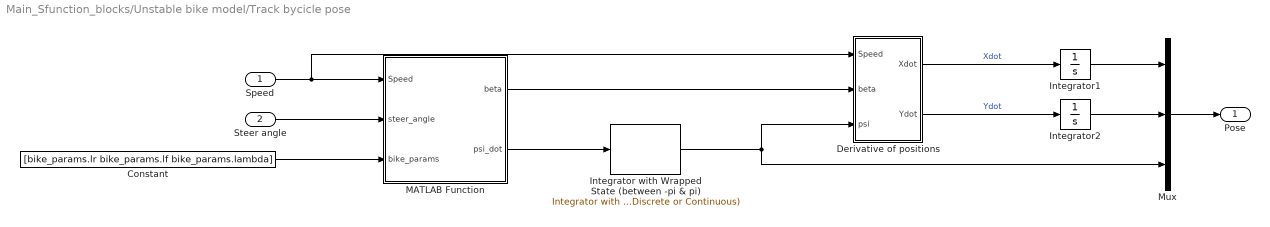
== system Main_Sfunction_blocks/Unstable bike model/Track bycicle pose ==
  Speed : Inport
  Steer angle : Inport  Port=2
  Constant : Constant  Value=[bike_params.lr bike_params.lf bike_params.lambda]
  Derivative of positions : MATLAB Function  TreatAsAtomicUnit=on
  Integrator with Wrapped State (between -pi & pi) : eeGeneralControl/Integrator with Wrapped State (Discrete or Continuous)  LabelModeActiveChoice=Discrete  WrappedStateUpperValue=pi  WrappedStateLowerValue=-pi  x0=initial_state.heading  Ts=Ts
  Integrator1 : Integrator  InitialCondition=initial_state.x
  Integrator2 : Integrator  InitialCondition=initial_state.y
  MATLAB Function : MATLAB Function  TreatAsAtomicUnit=on
  Mux : Mux  Inputs=3
  Pose : Outport
  wires:
  Derivative of positions/2(Ydot) -> Integrator2/1  "Ydot"
  Steer angle/1 -> MATLAB Function/2(steer_angle)
  Integrator2/1 -> Mux/2
  Mux/1 -> Pose/1
  Derivative of positions/1(Xdot) -> Integrator1/1  "Xdot"
  Speed/1 -> MATLAB Function/1(Speed), Derivative of positions/1(Speed)
  Integrator1/1 -> Mux/1
  MATLAB Function/1(beta) -> Derivative of positions/2(beta)
  Constant/1 -> MATLAB Function/3(bike_params)
  MATLAB Function/2(psi_dot) -> Integrator with Wrapped State (between -pi & pi)/1
  Integrator with Wrapped State (between -pi & pi)/1 -> Derivative of positions/3(psi), Mux/3

== matlab function Main_Sfunction_blocks/Unstable bike model/Nonlinear Bicycle model/MATLAB Function ==
  data: States input; xdot output; Steering_rate input; Speed input; disturbances input; bike_params input
function xdot = fcn(States, Steering_rate, Speed, disturbances, bike_params)
% Unpacked bike_params
    g = bike_params(1);
    h = bike_params(2);
    lr = bike_params(3);
    lf = bike_params(4);
    lambda = bike_params(5);
    c = bike_params(6);
    m = bike_params(7);
    h_imu = bike_params(8);

phi = States(1);%roll
delta = States(2);%steering angle
phi_d = States(3);%rollrate

% xdot = [phidot deltadot phiddot]
xdot1 = phi_d + disturbances(1);
xdot2 = Steering_rate + disturbances(2);
xdot3 = (g/h)*phi  + ((h*Speed^2-g*lr*c)/((lr+lf)*h^2))*delta*sin(lambda) + ((lr*Speed)/((lr+lf)*h))*Steering_rate*sin(lambda);

xdot = [xdot1 xdot2 xdot3]';

== matlab function Main_Sfunction_blocks/Unstable bike model/Track bycicle pose/Derivative of positions ==
  data: Speed input; beta input; psi input; Xdot output; Ydot output
function [Xdot, Ydot]  = fcn(Speed, beta, psi)

Xdot = Speed * cos(psi + beta);
Ydot = Speed * sin(psi + beta);

== matlab function Main_Sfunction_blocks/Unstable bike model/Nonlinear Bicycle model/Nonlinear Bicycle Model without front wheel inertia ==
  data: States input; Steering_rate input; Speed input; disturbances input; xdot output; Parameters parameter
function xdot = fcn(States, Steering_rate, Speed, disturbances, Parameters)

g = 9.81;

d_phidot = disturbances(1);
d_deltadot = disturbances(2);

phi = States(1);
delta = States(2);
phi_d = States(3);

% xdot = [phidot deltadot phiddot]
xdot1 = phi_d + d_phidot;
xdot2 = Steering_rate + d_deltadot;
xdot3 = (g/Parameters.h)*sin(phi) + ((Parameters.a*Speed)/(Parameters.b*Parameters.h))/(cos(sin(Parameters.lambda)*delta)^2)*sin(Parameters.lambda)*Steering_rate ...
                                  + ((Parameters.h*Speed^2-g*Parameters.a*Parameters.c)/(Parameters.b*Parameters.h^2))*sin(Parameters.lambda)*tan(delta);

xdot = [xdot1 xdot2 xdot3]';

== matlab function Main_Sfunction_blocks/Unstable bike model/Track bycicle pose/MATLAB Function ==
  data: Speed input; steer_angle input; beta output; bike_params input; psi_dot output
function [beta, psi_dot] = fcn(Speed, steer_angle, bike_params)
lr       = bike_params(1);
lf       = bike_params(2);
lambda  = bike_params(3);

eff_steering = steer_angle*sin(lambda);

beta = atan(lr /(lr+lf) * tan(eff_steering) );
psi_dot = (Speed / lr) * sin(beta);

== matlab function Main_Sfunction_blocks/Sensors/Define true sensor positions on the bike ==
  data: bike_params input; pose input; pose_corrected output
function pose_corrected  = fcn(bike_params, pose)
pose_corrected = pose;

gpsX = bike_params(1); % measured offset of GPS parallel to bike
gpsY = bike_params(2); % measured offset of GPS perpendicular to bike
gpsH = bike_params(3); % measured offset of GPS from ground to GPS

% define pose_l
pose_l = pose;

% Transform to local frame
    pose_l(1) =  pose(1) * cos(pose(3)) + pose(2) * sin(pose(3));
    pose_l(2) = -pose(1) * sin(pose(3)) + pose(2) * cos(pose(3)); 

% define actual positions of GPS 
% pose1 = difference in x in local frame
% pose2 = difference in y in local frame
    pose_l(1) = pose_l(1) + gpsX;
    pose_l(2) = pose_l(2) + gpsY + gpsH*sin(pose(4));

% define actual positions of IMU 


% Transform back to global frame
    pose(1) = pose_l(1) * cos(pose(3)) - pose_l(2) * sin(pose(3));
    pose(2) = pose_l(1) * sin(pose(3)) + pose_l(2) * cos(pose(3));

pose_corrected(1) = pose(1);
pose_corrected(2) = pose(2);
